simulink library "NullAircraftStateRateBus"  (R2018b)
settings: Solver=VariableStepAuto  StartTime=0.0  StopTime=10.0  RelTol=1e-3
settings Model: Creator=RA24876  LastModifiedBy=RA24876
settings SFSimCC: SimUseLocalCustomCode=off
settings RTWCC: RTWUseLocalCustomCode=off
settings CodeAppCC: StateflowObjectComments=on

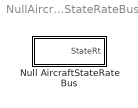
== system NullAircraftStateRateBus ==
  Null AircraftStateRate Bus : Subsystem  mask(Null AircraftStateRate Bus){}
      mask help: Creates an AircraftStateRate bus signal with all null values. Assign values to elements with a Bus Assignment block.

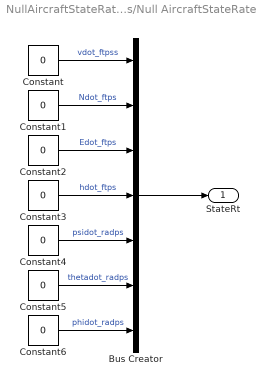
== system NullAircraftStateRateBus/Null AircraftStateRate Bus ==
  Bus Creator : BusCreator  Inputs=7  OutDataTypeStr=Bus: AircraftStateRate
      settings: InheritFromInputs=off
  Constant{,1..6} (7 alike) : Constant  Value=0
  StateRt : Outport  OutDataTypeStr=Bus: AircraftStateRate
  wires:
  Constant6/1 -> Bus Creator/7  "phidot_radps"
  Constant2/1 -> Bus Creator/3  "Edot_ftps"
  Constant/1 -> Bus Creator/1  "vdot_ftpss"
  Constant3/1 -> Bus Creator/4  "hdot_ftps"
  Constant5/1 -> Bus Creator/6  "thetadot_radps"
  Constant4/1 -> Bus Creator/5  "psidot_radps"
  Bus Creator/1 -> StateRt/1
  Constant1/1 -> Bus Creator/2  "Ndot_ftps"
